simulink model "TCS_fuzzy_logic implementation"  (R2020b)
settings: Solver=FixedStepAuto  StartTime=0.0  StopTime=inf  RelTol=1e-3  EnableMultiTasking=on
libraries: arduinolib x2, fuzblock x1
settings Model: SILPILModeSetting=veronly  ExtModeTrigDuration=2  Creator=roman  LastModifiedBy=roman
settings SolverCC: AutoInsertRateTranBlk=on
settings OptimizationCC: EnhancedBackFolding=on  PassReuseOutputArgsAs=Individual arguments  ZeroExternalMemoryAtStartup=off  ZeroInternalMemoryAtStartup=off  MaxStackSize=64  OptimizeBlockOrder=speed  DifferentSizesBufferReuse=on  OptimizationCustomize=off  EfficientTunableParamExpr=on
settings DebuggingCC: ParameterTunabilityLossMsg=error
settings HardwareCC: ProdBitPerInt=16  ProdBitPerPointer=16  ProdBitPerSizeT=16  ProdBitPerPtrDiffT=16  ProdLargestAtomicFloat=None  ProdWordSize=8  ProdHWDeviceType=Atmel->AVR
settings SFSimCC: MATLABDynamicMemAlloc=off
settings RTWCC: Description=Embedded Coder  SystemTargetFile=ert.tlc  HardwareBoard=Arduino Uno  TemplateMakefile=ert_default_tmf  Toolchain=Arduino AVR  BuildConfiguration=Faster Runs
settings CodeAppCC: ForceParamTrailComments=on  IgnoreCustomStorageClasses=off  OperatorAnnotations=on  SimulinkDataObjDesc=on  SFDataObjDesc=on  InsertBlockDesc=on
settings ERTTargetCC: SupportContinuousTime=on  SupportVariableSizeSignals=on  ExtModeStaticAllocSize=250

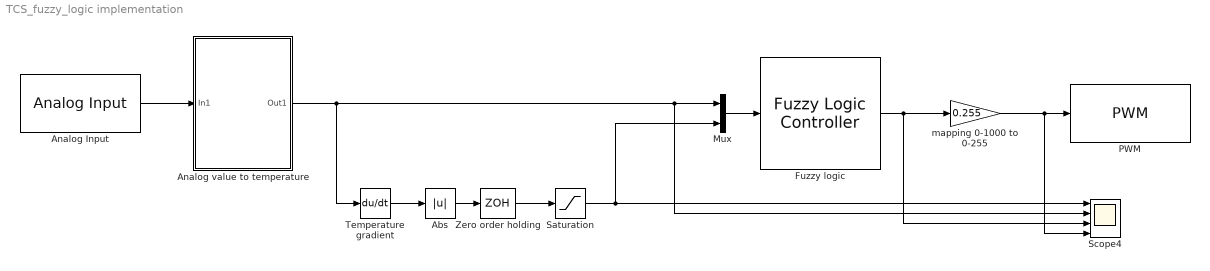
== system TCS_fuzzy_logic implementation ==
  Abs : Abs
  Analog Input : arduinolib/Analog Input  pinNumber=0  ReadResultsOnly=off  ConversionTriggerSource=Software  ExternalTriggerType=uint32( 0 )  OutputDataType=uint16  EnableConversionCompleteNotify=off  EnableOuputStatus=off  SampleTime=30  blockPlatform=arduino
  Analog value to temperature : Subsystem
  Fuzzy logic : fuzblock/Fuzzy Logic  Controller  FIS=fuzzy  OutputSampleNumber=101  DataType=double  FuzzifiedInputs=off  RuleFiringStrengths=off  RuleOutputs=off  AggregatedOutputs=off  SimulateUsing=Interpreted execution  OutOfRangeInputValueMessage=warning  NoRuleFiredMessage=warning  EmptyOutputFuzzySetMessage=warning
  Mux : Mux  Inputs=2
  PWM : arduinolib/PWM  pinNumber=10  frequencyType=Default  desiredFrequency=490.2  achievableFrequency=490.2
  Saturation : Saturate  UpperLimit=0.01  LowerLimit=0.0001
  Scope4 : Scope  NumInputPorts=4
  Temperature gradient : Derivative
  Zero order holding : ZeroOrderHold  SampleTime=3600
  mapping 0-1000 to 0-255 : Gain  Gain=0.255
  wires:
  Mux/1 -> Fuzzy logic/1
  mapping 0-1000 to 0-255/1 -> Scope4/4, PWM/1
  Fuzzy logic/1 -> Scope4/3, mapping 0-1000 to 0-255/1
  Temperature gradient/1 -> Abs/1
  Analog value to temperature/1(Out1) -> Temperature gradient/1, Scope4/2, Mux/1
  Analog Input/1 -> Analog value to temperature/1(In1)
  Abs/1 -> Zero order holding/1
  Saturation/1 -> Mux/2, Scope4/1
  Zero order holding/1 -> Saturation/1

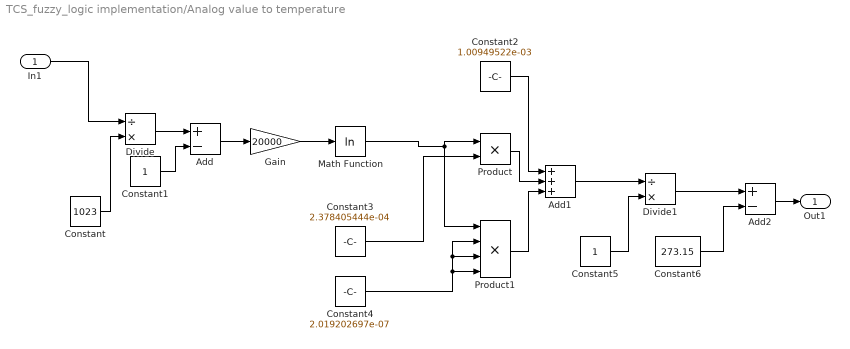
== system TCS_fuzzy_logic implementation/Analog value to temperature ==
  In1 : Inport
  Add : Sum  Inputs=+-
  Add1 : Sum  Inputs=+++  OutDataTypeStr=double
  Add2 : Sum  Inputs=+-
  Constant : Constant  Value=1023
  Constant1 : Constant
  Constant2 : Constant  Value=1.00949522e-03  OutDataTypeStr=double
  Constant3 : Constant  Value=2.378405444e-04  OutDataTypeStr=double
  Constant4 : Constant  Value=2.019202697e-07  OutDataTypeStr=double
  Constant5 : Constant  OutDataTypeStr=double
  Constant6 : Constant  Value=273.15
  Divide : Product  Inputs=/*
  Divide1 : Product  Inputs=/*  OutDataTypeStr=double
  Gain : Gain  Gain=20000
  Math Function : Math  Operator=log  SaturateOnIntegerOverflow=on
  Product : Product  OutDataTypeStr=double
  Product1 : Product  Inputs=4  OutDataTypeStr=double
  Out1 : Outport
  wires:
  Constant3/1 -> Product/2
  Product/1 -> Add1/2
  Constant1/1 -> Add/2
  Constant6/1 -> Add2/2
  Divide/1 -> Add/1
  Constant/1 -> Divide/2
  Constant4/1 -> Product1/4, Product1/3, Product1/2
  Add2/1 -> Out1/1
  Add/1 -> Gain/1
  Math Function/1 -> Product1/1, Product/1
  Product1/1 -> Add1/3
  Add1/1 -> Divide1/1
  Divide1/1 -> Add2/1
  Constant5/1 -> Divide1/2
  Gain/1 -> Math Function/1
  Constant2/1 -> Add1/1
  In1/1 -> Divide/1
